simulink model "spiking_neuron"  (R2022a)
settings: Solver=FixedStepAuto  StartTime=0.0  StopTime=100  FixedStep=0.05  RelTol=1e-3
values from neighbouring files (symbols this model uses):
  u0 = x0(i,2)    [gen_data.m]
  v0 = x0(i,1)-63    [gen_data.m]
settings Model: Creator=diego  LastModifiedBy=diego

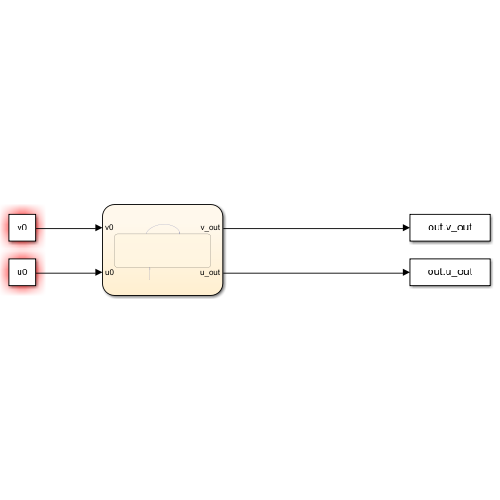
[thumbnail: Simulink's stored preview of the top-level diagram]
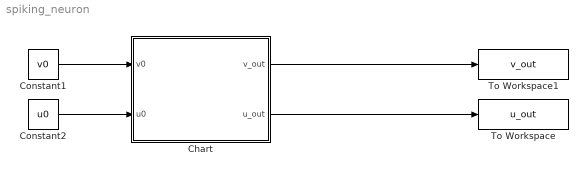
== system spiking_neuron ==
  Chart : Stateflow chart  TreatAsAtomicUnit=on
  Constant1 : Constant  Value=v0
  Constant2 : Constant  Value=u0
  To Workspace : ToWorkspace  VariableName=u_out  SampleTime=-1
  To Workspace1 : ToWorkspace  VariableName=v_out  SampleTime=-1
  wires:
  Chart/1(v_out) -> To Workspace1/1
  Chart/2(u_out) -> To Workspace/1
  Constant1/1 -> Chart/1(v0)
  Constant2/1 -> Chart/2(u0)

== stateflow chart spiking_neuron/Chart ==
  settings: updateMethod=CONTINUOUS
  state Mode1
    du:
    v_dot = 0.04*v^2 + 5*v + 140 - u + 40;
    u_dot = 0.02*(0.2*v-u);
    v_out = v;
    u_out = u;
  Mode1 -> Mode1 : [v > 30]{v = -65; u = u+8;}
  (default) -> Mode1 : {v = v0;
      | u = u0;}
  data: v_out output; u_out output; v local; u local; v0 input; u0 input
  data v settings: updateMethod=SF_CONTINUOUS_TIME_DATA
  data u settings: updateMethod=SF_CONTINUOUS_TIME_DATA
